simulink model "three_phase_bridge_inverter_2"  (R2017a)
settings: Solver=VariableStepAuto  StartTime=0.0  StopTime=0.1  MaxStep=1e-4  RelTol=1e-3
libraries: powerlib x14, powerlib_meascontrol x4, powerlib_extras x1
settings Model: Creator=Administrator  LastModifiedBy=Administrator

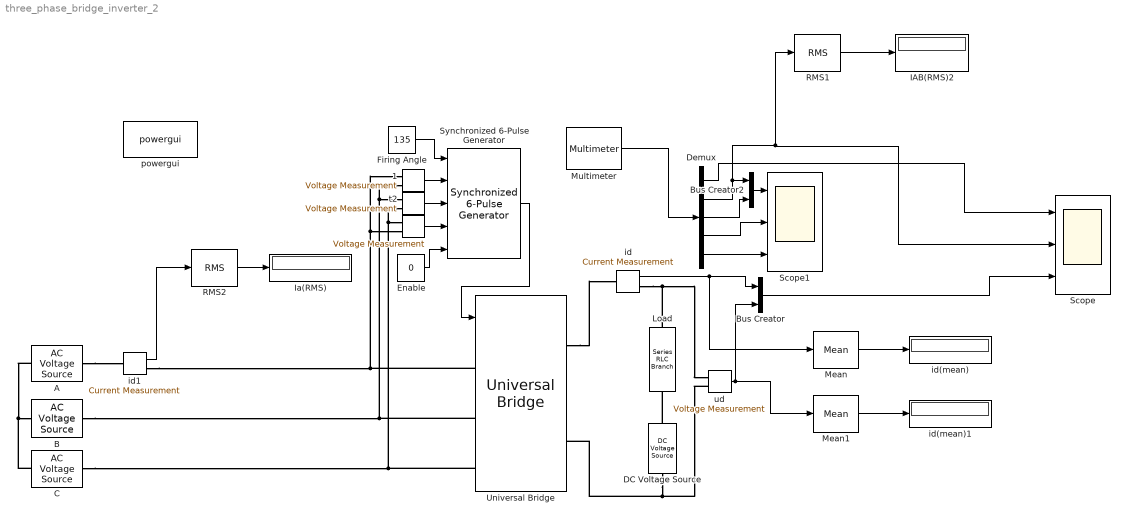
== system three_phase_bridge_inverter_2 ==
  " " : powerlib/Measurements/Voltage Measurement  PhasorSimulation=off  OutputType=Complex  PSBequivalent=0
  1 : powerlib/Measurements/Voltage Measurement  PhasorSimulation=off  OutputType=Complex  PSBequivalent=0
  A : powerlib/Electrical Sources/AC Voltage Source  Amplitude=311  Phase=30  Frequency=50  SampleTime=0  Measurements=None  BusType=swing  Pref=10e3  Qref=0  Qmin=-inf  Qmax=+inf
  B : powerlib/Electrical Sources/AC Voltage Source  Amplitude=311  Phase=-90  Frequency=50  SampleTime=0  Measurements=None  BusType=swing  Pref=10e3  Qref=0  Qmin=-inf  Qmax=+inf
  Bus Creator : BusCreator  DialogController=Simulink.DDGSource_Bus  Inputs=2
  Bus Creator2 : BusCreator  DialogController=Simulink.DDGSource_Bus  Inputs=2
  C : powerlib/Electrical Sources/AC Voltage Source  Amplitude=311  Phase=-210  Frequency=50  SampleTime=0  Measurements=None  BusType=swing  Pref=10e3  Qref=0  Qmin=-inf  Qmax=+inf
  DC Voltage Source : powerlib/Electrical Sources/DC Voltage Source  Amplitude=500  Measurements=None
  Demux : Demux  Outputs=5
  Enable : Constant  Value=0
  Firing Angle : Constant  Value=135
  IAB(RMS)2 : Display
  Ia(RMS) : Display
  Load : powerlib/Elements/Series RLC Branch  LConnTagsString=__new0  RConnTagsString=__new0  BranchType=RLC  Resistance=2  Inductance=0.02  SetiL0=off  InitialCurrent=0  Capacitance=0  Setx0=off  InitialVoltage=0  Measurements=Branch voltage and current
  Mean : powerlib_meascontrol/Measurements/Mean  Freq=60  Vinit=0  Ts=0
  Mean1 : powerlib_meascontrol/Measurements/Mean  Freq=60  Vinit=0  Ts=0
  Multimeter : powerlib/Measurements/Multimeter  Tag=PoWeRsYsTeMmEaSuReMeNt  PhasorSimulation=off  OutputType=Magnitude  sel=[2 13 16 14 18]  L=18  Gain=[1 1 1 1 1]  yselected={'Usw1: Universal Bridge','Isw1: Universal Bridge','Isw4: Universal Bridge','Isw2: Universal Bridge','Isw6: Universal Bridge'};  PSBOutputType=1  PSBequivalent=0  AxesSetting=[0,0.1,-100,100]  Display=0  SavedBlockNames=-11
      settings: AttributesFormatString=\n
  RMS1 : powerlib_meascontrol/Measurements/RMS  TrueRMS=on  Freq=60  RMSInit=0  Ts=0
  RMS2 : powerlib_meascontrol/Measurements/RMS  TrueRMS=on  Freq=60  RMSInit=120  Ts=0
  Scope : Scope  NumInputPorts=3
  Scope1 : Scope  NumInputPorts=3
  Synchronized 6-Pulse Generator : powerlib_extras/Control  Blocks/Synchronized 6-Pulse Generator  freq=50  pwidth=10  Double_Pulse=on
  Universal Bridge : powerlib/Power Electronics/Universal Bridge  Arms=3  SnubberResistance=1e5  SnubberCapacitance=inf  Device=Thyristors  Ron=1e-3  Lon=0  ForwardVoltages="[  0  0  ]"  ForwardVoltage=0  GTOparameters=[ 10e-6 , 20e-6 ]  IGBTparameters=[ 1e-6 , 2e-6 ]  Measurements=All voltages and currents  Measurements_2=None  converterType=Rectifier
  id : powerlib/Measurements/Current Measurement  PhasorSimulation=off  OutputType=Complex  PSBequivalent=0
  id(mean) : Display
  id(mean)1 : Display
  id1 : powerlib/Measurements/Current Measurement  PhasorSimulation=off  OutputType=Complex  PSBequivalent=0
  powergui : powerlib/powergui  Priority=1  SimulationMode=Continuous  SampleTime=50e-6  frequency=60  Iterations=50  frequencyindice=50  Pbase=100e6  ErrMax=1e-4  UnitsV=kV  UnitsW=MW  buscounter=0  FunctionMessages=off  echomessages=off  EnableUseOfTLC=off  CurrentSourceSwitches=off  DisableSnubberDevices=off  DisableRonSwitches=off  DisableVfSwitches=off  DisplayEquations=off  SolverType=Tustin/Backward Euler (TBE)  Interpol=off  ExternalGateDelay=off  methode=off  Ts=100  x0status=blocks  SPID=on  SwTol=0  HookPort=off  RestoreLinks=warning  ResistiveCurrentMeasurement=off  Frange=[0:2:500]  Ylog=off  Xlog=on  ShowGrid=off  save=off  variable=ZData  structure=0  ZoomFFT=off  StartTime=0.0  cycles=1  DisplayStyle=1  fundamental=60  FreqAxis=off  MaxFrequency=1000  frequencyindicesteady=1  RmsSteady=1  display=off
  t2 : powerlib/Measurements/Voltage Measurement  PhasorSimulation=off  OutputType=Complex  PSBequivalent=0
  ud : powerlib/Measurements/Voltage Measurement  PhasorSimulation=off  OutputType=Complex  PSBequivalent=0
  wires:
  Enable/1 -> Synchronized 6-Pulse Generator/5
  1/1 -> Synchronized 6-Pulse Generator/2
  " "/1 -> Synchronized 6-Pulse Generator/4
  t2/1 -> Synchronized 6-Pulse Generator/3
  Firing Angle/1 -> Synchronized 6-Pulse Generator/1
  Synchronized 6-Pulse Generator/1 -> Universal Bridge/1
  Bus Creator/1 -> Scope/3
  ud/1 -> Mean1/1, Bus Creator/2
  id/1 -> Mean/1, Bus Creator/1
  Mean/1 -> id(mean)/1
  id1/1 -> RMS2/1
  RMS2/1 -> Ia(RMS)/1
  Multimeter/1 -> Demux/1
  Demux/4 -> Scope1/2
  Demux/3 -> Bus Creator2/2
  Bus Creator2/1 -> Scope1/1
  Demux/5 -> Scope1/3
  Demux/1 -> Scope/1
  Mean1/1 -> id(mean)1/1
  Demux/2 -> Scope/2, RMS1/1, Bus Creator2/1
  RMS1/1 -> IAB(RMS)2/1
  connections:
  " "/LConn2 -- Universal Bridge/LConn1 -- id1/RConn1 -- 1/LConn1
  Load/LConn1 -- id/RConn1 -- ud/LConn1
  " "/LConn1 -- Universal Bridge/LConn3 -- C/RConn1 -- t2/LConn2
  DC Voltage Source/RConn1 -- ud/LConn2 -- Universal Bridge/RConn2
  Universal Bridge/LConn2 -- B/RConn1 -- 1/LConn2 -- t2/LConn1
  B/LConn1 -- C/LConn1 -- A/LConn1
  Universal Bridge/RConn1 -- id/LConn1
  DC Voltage Source/LConn1 -- Load/RConn1
  A/RConn1 -- id1/LConn1
